simulink model "ScriptDemo"  (R2022b)
settings: configuration reference "TmVcThermal_Configuration_sub" (kept outside this file)
undefined symbols (not defined in the file): aaaa, bbbb, cTmComprCtrl_D_u8HvacFlowTable_db, cTmComprCtrl_D_u8HvacFlowTable_sw, cTmComprCtrl_n_i16ChillCmpIMax, cTmComprCtrl_n_i16ChillCmpIMin, cTmComprCtrl_n_i16ChillCmpIMin666, cTmComprCtrl_n_i16ChillCmpPMax, cTmComprCtrl_n_i16ChillCmpPMin, cTmComprCtrl_n_i16CmpChillCoolRpmKiMax, cTmComprCtrl_n_i16CmpChillCoolRpmKiMin, cTmComprCtrl_n_i16CmpChillCoolRpmKpMax, cTmComprCtrl_n_i16CmpChillCoolRpmKpMin, cTmComprCtrl_n_i16CmpCoolRpmKiMax, cTmComprCtrl_n_i16CmpCoolRpmKiMin, cTmComprCtrl_n_i16CmpCoolRpmKpMax, cTmComprCtrl_n_i16CmpCoolRpmKpMin, cTmComprCtrl_n_i16SM4CmpHeatKiMax, cTmComprCtrl_n_i16SM4CmpHeatKiMin, cTmComprCtrl_n_i16SM4CmpHeatKpMax, cTmComprCtrl_n_i16SM4CmpHeatKpMin, cTmComprCtrl_n_i16SM5CmpHeatKiMax, cTmComprCtrl_n_i16SM5CmpHeatKiMin, cTmComprCtrl_n_i16SM5CmpHeatKpMax, cTmComprCtrl_n_i16SM5CmpHeatKpMin, cTmComprCtrl_n_i16SM6CmpHeatKiMax, cTmComprCtrl_n_i16SM6CmpHeatKiMin, cTmComprCtrl_n_i16SM6CmpHeatKpMax, cTmComprCtrl_n_i16SM6CmpHeatKpMin, cTmComprCtrl_n_u16CmpMaxSpdFanFltLimt, cTmComprCtrl_n_u16CmpMaxSpdLoSidePFltLimt, cTmComprCtrl_n_u16CmpMaxSpdSensorFltLimt, cTmComprCtrl_n_u16CompMinRpm, cTmComprCtrl_n_u16CompRpmIncThres, cTmComprCtrl_t_u16BattCooltFFPeriod, cTmComprCtrl_t_u16BattCooltPIPeriod, cTmComprCtrl_t_u16CmpCoolFFPeriod, cTmComprCtrl_t_u16CmpCoolPIPeriod, cTmComprCtrl_t_u16CoolCmpChillFFPeriod, cTmComprCtrl_t_u16CoolCmpChillPIPeriod, cTmComprCtrl_t_u16SM4CmpHeatFFPeriod, cTmComprCtrl_t_u16SM4CmpHeatPIPeriod, cTmComprCtrl_t_u16SM5CmpHeatFFPeriod, cTmComprCtrl_t_u16SM5CmpHeatPIPeriod, cTmComprCtrl_t_u16SM6CmpHeatFFPeriod, cTmComprCtrl_t_u16SM6CmpHeatPIPeriod, cTmComprCtrl_Te_EvapClearInteg, cTmComprCtrl_Te_i16HpReqTempSaturoffset, cTmComprCtrl_Te_i16SatLpReplaceDiff, cTmComprCtrl_Te_i16SM3BatDiffStartEvapDecOffset, cTmComprCtrl_Te_i16SM3EvapLo, cTmComprCtrl_Te_i16SM3TBatDiffEntEvapDecOffset, cTmComprCtrl_Te_i16SM3TBatDiffEntEvapDecOffsetQuit, cTmComprCtrl_Te_s32ErrCmpChillPIContinueCoolH, cTmComprCtrl_Te_s32ErrCmpChillPIContinueCoolL, cTmComprCtrl_Te_s32ErrCmpPIContinueChillH, cTmComprCtrl_Te_s32ErrCmpPIContinueChillL, cTmComprCtrl_Te_s32ErrCmpPIContinueCoolH, cTmComprCtrl_Te_s32ErrCmpPIContinueCoolL, cTmComprCtrl_Te_s32ErrCmpPIContinueHeatH ... (+398)
libraries: simulink x782, PCMULib x640, simulink_need_slupdate x4
(part 14 of 41)

== system ScriptDemo/Create/createMerge/Before/ID29332_RpmPI ==
  note: 测试步骤：
      | 使能测试
      | 清I测试
      | 	不使能
      | 	模式切换
      | 保持I测试
      | 	上限保持
      | 	下限保持
      | 	边界限制清I保持
      | 累计限值
      | 	累计Kp, Ki 上限
      | 	累计Kp, Ki 下限
      | 正常PI测试
      | 	上升
      | 	下降
  rTmComprCtrl_Te_s32LowErrStop : Inport  OutDataTypeStr=single
  rTmComprCtrl_Te_s32TempError : Inport  Port=2  OutDataTypeStr=single
  rTmComprCtrl_Te_s32UpErrStop : Inport  Port=3  OutDataTypeStr=single
  rTmComprCtrl_n_u16ComprRpmFF : Inport  Port=4  OutDataTypeStr=uint16
  rTmComprCtrl_n_u16ComprRpmKi : Inport  Port=5  OutDataTypeStr=uint16
  rTmComprCtrl_n_u16ComprRpmKp : Inport  Port=6  OutDataTypeStr=uint16
  rTmComprCtrl_n_u16DisOverrideValue : Inport  Port=7  OutDataTypeStr=uint16
  rTmComprCtrl_n_i16KiLowLimit : Inport  Port=8  OutDataTypeStr=int16
  rTmComprCtrl_n_i16KiUpLimit : Inport  Port=9  OutDataTypeStr=int16
  rTmComprCtrl_n_i16KpLowLimit : Inport  Port=10  OutDataTypeStr=int16
  rTmComprCtrl_n_i16KpUpLimit : Inport  Port=11  OutDataTypeStr=int16
  rTmComprCtrl_t_u16PIPeriod : Inport  Port=12  OutDataTypeStr=uint16
  xTmComprCtrl_B_CompOnReqCompOn : Inport  Port=13  OutDataTypeStr=boolean
  xTmComprCtrl_B_Enable : Inport  Port=14  OutDataTypeStr=boolean
  xTmComprCtrl_B_ModeChanged : Inport  Port=15  OutDataTypeStr=boolean
  xTmComprCtrl_B_ReduceRpm : Inport  Port=16  OutDataTypeStr=boolean
  sTmRefriModeMgr_D_u8HPCurMode : Inport  Port=17  OutDataTypeStr=uint8
  sTmSigProces_Te_s32EvapFanFilter : Inport  Port=18  OutDataTypeStr=single
  yTmRefriModeMgr_B_CoolModeInCycle : Inport  Port=19  OutDataTypeStr=boolean
  yTmRefriModeMgr_B_HeatModeInCycle : Inport  Port=20  OutDataTypeStr=boolean
  ClearInteg : Subsystem  TreatAsAtomicUnit=on
  IndebugRvs : PCMULib/Interface/IndebugRvs  SWI=cTmComprCtrl_Te_s32LowErrStop_swi  DBI=cTmComprCtrl_Te_s32LowErrStop_dbi
      settings: SourceProductName=PCMULib
  IndebugRvs1 : PCMULib/Interface/IndebugRvs  SWI=cTmComprCtrl_Te_s32TempError_swi  DBI=cTmComprCtrl_Te_s32TempError_dbi
      settings: SourceProductName=PCMULib
  IndebugRvs10 : PCMULib/Interface/IndebugRvs  SWI=cTmComprCtrl_n_i16KpUpLimit_swi  DBI=cTmComprCtrl_n_i16KpUpLimit_dbi
      settings: SourceProductName=PCMULib
  IndebugRvs11 : PCMULib/Interface/IndebugRvs  SWI=cTmComprCtrl_t_u16PIPeriod_swi  DBI=cTmComprCtrl_t_u16PIPeriod_dbi
      settings: SourceProductName=PCMULib
  IndebugRvs12 : PCMULib/Interface/IndebugRvs  SWI=cTmComprCtrl_B_Enable_swi  DBI=cTmComprCtrl_B_Enable_dbi
      settings: SourceProductName=PCMULib
  IndebugRvs13 : PCMULib/Interface/IndebugRvs  SWI=cTmComprCtrl_B_ModeChanged_swi  DBI=cTmComprCtrl_B_ModeChanged_dbi
      settings: SourceProductName=PCMULib
  IndebugRvs2 : PCMULib/Interface/IndebugRvs  SWI=cTmComprCtrl_Te_s32UpErrStop_swi  DBI=cTmComprCtrl_Te_s32UpErrStop_dbi
      settings: SourceProductName=PCMULib
  IndebugRvs3 : PCMULib/Interface/IndebugRvs  SWI=cTmComprCtrl_n_u16ComprRpmFF_swi  DBI=cTmComprCtrl_n_u16ComprRpmFF_dbi
      settings: SourceProductName=PCMULib
  IndebugRvs4 : PCMULib/Interface/IndebugRvs  SWI=cTmComprCtrl_n_u16ComprRpmKi_swi  DBI=cTmComprCtrl_n_u16ComprRpmKi_dbi
      settings: SourceProductName=PCMULib
  IndebugRvs5 : PCMULib/Interface/IndebugRvs  SWI=cTmComprCtrl_n_u16ComprRpmKp_swi  DBI=cTmComprCtrl_n_u16ComprRpmKp_dbi
      settings: SourceProductName=PCMULib
  IndebugRvs6 : PCMULib/Interface/IndebugRvs  SWI=cTmComprCtrl_n_u16DisOverrideValue_swi  DBI=cTmComprCtrl_n_u16DisOverrideValue_dbi
      settings: SourceProductName=PCMULib
  IndebugRvs7 : PCMULib/Interface/IndebugRvs  SWI=cTmComprCtrl_n_i16KiLowLimit_swi  DBI=cTmComprCtrl_n_i16KiLowLimit_dbi
      settings: SourceProductName=PCMULib
  IndebugRvs8 : PCMULib/Interface/IndebugRvs  SWI=cTmComprCtrl_n_i16KiUpLimit_swi  DBI=cTmComprCtrl_n_i16KiUpLimit_dbi
      settings: SourceProductName=PCMULib
  IndebugRvs9 : PCMULib/Interface/IndebugRvs  SWI=cTmComprCtrl_n_i16KpLowLimit_swi  DBI=cTmComprCtrl_n_i16KpLowLimit_dbi
      settings: SourceProductName=PCMULib
  PIControler : Subsystem  AncestorBlock=PCMULib/Calculation/PI
  rTmComprCtrl_n_u16CompRpmReqPI : Outport  OutDataTypeStr=uint16
  wires:
  [rTmComprCtrl_t_u16PIPeriod] -> PIControler/3(rTmComprCtrl_t_u16PIPeriod)
  [rTmComprCtrl_Te_s32TempError] -> PIControler/4(rTmComprCtrl_Te_s32TempError)
  [rTmComprCtrl_n_u16ComprRpmFF] -> PIControler/5(rTmComprCtrl_n_u16ComprRpmFF)
  [rTmComprCtrl_n_u16ComprRpmKp] -> PIControler/6(rTmComprCtrl_n_u16ComprRpmKp)
  [rTmComprCtrl_n_u16ComprRpmKi] -> PIControler/7(rTmComprCtrl_n_u16ComprRpmKi)
  [rTmComprCtrl_n_i16KpLowLimit] -> PIControler/9(rTmComprCtrl_n_i16KpLowLimit)
  [rTmComprCtrl_n_i16KiUpLimit] -> PIControler/10(rTmComprCtrl_n_i16KiUpLimit)
  [rTmComprCtrl_n_i16KiLowLimit] -> PIControler/11(rTmComprCtrl_n_i16KiLowLimit)
  [rTmComprCtrl_Te_s32UpErrStop] -> PIControler/12(rTmComprCtrl_Te_s32UpErrStop)
  [rTmComprCtrl_Te_s32LowErrStop] -> PIControler/13(rTmComprCtrl_Te_s32LowErrStop)
  [rTmComprCtrl_n_u16DisOverrideValue] -> PIControler/14(rTmComprCtrl_n_u16DisOverrideValue)
  PIControler/1(rPIControler_n_u16CompRpmReq) -> [rPIControler_n_u16CompRpmReq]
  rTmComprCtrl_Te_s32LowErrStop/1 -> IndebugRvs/1
  rTmComprCtrl_Te_s32TempError/1 -> IndebugRvs1/1
  rTmComprCtrl_Te_s32UpErrStop/1 -> IndebugRvs2/1
  rTmComprCtrl_n_u16ComprRpmFF/1 -> IndebugRvs3/1
  rTmComprCtrl_n_u16ComprRpmKi/1 -> IndebugRvs4/1
  rTmComprCtrl_n_u16ComprRpmKp/1 -> IndebugRvs5/1
  rTmComprCtrl_n_u16DisOverrideValue/1 -> IndebugRvs6/1
  rTmComprCtrl_n_i16KiLowLimit/1 -> IndebugRvs7/1
  rTmComprCtrl_n_i16KiUpLimit/1 -> IndebugRvs8/1
  rTmComprCtrl_n_i16KpLowLimit/1 -> IndebugRvs9/1
  rTmComprCtrl_n_i16KpUpLimit/1 -> IndebugRvs10/1
  rTmComprCtrl_t_u16PIPeriod/1 -> IndebugRvs11/1
  xTmComprCtrl_B_CompOnReqCompOn/1 -> [xTmComprCtrl_B_CompOnReqCompOn]
  [rPIControler_n_u16CompRpmReq] -> rTmComprCtrl_n_u16CompRpmReqPI/1
  xTmComprCtrl_B_Enable/1 -> IndebugRvs12/1
  xTmComprCtrl_B_ModeChanged/1 -> IndebugRvs13/1
  IndebugRvs/1 -> [rTmComprCtrl_Te_s32LowErrStop]  "rTmComprCtrl_Te_s32LowErrStop"
  IndebugRvs1/1 -> [rTmComprCtrl_Te_s32TempError]  "rTmComprCtrl_Te_s32TempError"
  IndebugRvs2/1 -> [rTmComprCtrl_Te_s32UpErrStop]  "rTmComprCtrl_Te_s32UpErrStop"
  IndebugRvs3/1 -> [rTmComprCtrl_n_u16ComprRpmFF]  "rTmComprCtrl_n_u16ComprRpmFF"
  IndebugRvs4/1 -> [rTmComprCtrl_n_u16ComprRpmKi]  "rTmComprCtrl_n_u16ComprRpmKi"
  IndebugRvs5/1 -> [rTmComprCtrl_n_u16ComprRpmKp]  "rTmComprCtrl_n_u16ComprRpmKp"
  IndebugRvs7/1 -> [rTmComprCtrl_n_i16KiLowLimit]  "rTmComprCtrl_n_i16KiLowLimit"
  IndebugRvs6/1 -> [rTmComprCtrl_n_u16DisOverrideValue]  "rTmComprCtrl_n_u16DisOverrideValue"
  IndebugRvs8/1 -> [rTmComprCtrl_n_i16KiUpLimit]  "rTmComprCtrl_n_i16KiUpLimit"
  IndebugRvs9/1 -> [rTmComprCtrl_n_i16KpLowLimit]  "rTmComprCtrl_n_i16KpLowLimit"
  IndebugRvs11/1 -> [rTmComprCtrl_t_u16PIPeriod]  "rTmComprCtrl_t_u16PIPeriod"
  IndebugRvs10/1 -> [rTmComprCtrl_n_i16KpUpLimit]  "rTmComprCtrl_n_i16KpUpLimit"
  IndebugRvs12/1 -> [xTmComprCtrl_B_Enable]  "xTmComprCtrl_B_Enable"
  IndebugRvs13/1 -> [xTmComprCtrl_B_ModeChanged]  "xTmComprCtrl_B_ModeChanged"
  xTmComprCtrl_B_ReduceRpm/1 -> [xTmComprCtrl_B_ReduceRpm]
  [xTmComprCtrl_B_ReduceRpm] -> PIControler/15(xTmComprCtrl_B_ReduceRpm)
  [rTmComprCtrl_n_i16KpUpLimit] -> PIControler/8(rTmComprCtrl_n_i16KpUpLimit)
  [xTmComprCtrl_B_Enable] -> PIControler/1(xTmComprCtrl_B_Enable)
  PIControler/2(rPIControler_n_s32SAccmKi) -> [rPIControler_n_s32SAccmKi]
  [rPIControler_n_s32SAccmKi] -> ClearInteg/1(rPIControler_n_s32SAccmKi)
  [sTmRefriModeMgr_D_u8HPCurMode] -> ClearInteg/2(sTmRefriModeMgr_D_u8HPCurMode)
  [sTmSigProces_Te_s32EvapFanFilter] -> ClearInteg/3(sTmSigProces_Te_s32EvapFanFilter)
  [xTmComprCtrl_B_CompOnReqCompOn] -> ClearInteg/4(xTmComprCtrl_B_CompOnReqCompOn)
  [xTmComprCtrl_B_ModeChanged] -> ClearInteg/5(xTmComprCtrl_B_ModeChanged)
  ClearInteg/1(xClearInteg_B_ClearInteg) -> [xClearInteg_B_ClearInteg]
  [xClearInteg_B_ClearInteg] -> PIControler/2(xTmComprCtrl_B_ClearInteg)
  sTmRefriModeMgr_D_u8HPCurMode/1 -> [sTmRefriModeMgr_D_u8HPCurMode]
  sTmSigProces_Te_s32EvapFanFilter/1 -> [sTmSigProces_Te_s32EvapFanFilter]
  [yTmRefriModeMgr_B_CoolModeInCycle] -> ClearInteg/6(yTmRefriModeMgr_B_CoolModeInCycle)
  [yTmRefriModeMgr_B_HeatModeInCycle] -> ClearInteg/7(yTmRefriModeMgr_B_HeatModeInCycle)
  yTmRefriModeMgr_B_CoolModeInCycle/1 -> [yTmRefriModeMgr_B_CoolModeInCycle]
  yTmRefriModeMgr_B_HeatModeInCycle/1 -> [yTmRefriModeMgr_B_HeatModeInCycle]

== system ScriptDemo/Create/createMerge/Before/SM0 ==
  Action Port : ActionPort
  Constant{,1..2,10} (4 alike) : Constant  Value=0  OutDataTypeStr=uint16
  Constant11 : Constant  Value=5  OutDataTypeStr=uint16
  Constant12 : Constant  Value=0  OutDataTypeStr=boolean
  Constant3 : Constant  Value=0  OutDataTypeStr=single
  Constant4 : Constant  Value=0  OutDataTypeStr=single
  Constant5 : Constant  Value=0  OutDataTypeStr=single
  Constant{6..9} (4 alike) : Constant  Value=0  OutDataTypeStr=int16
  rSM0_Te_s32TempError : Outport  OutDataTypeStr=single
  rSM0_n_u16ComprRpmFF : Outport  Port=2  OutDataTypeStr=uint16
  rSM0_n_u16DisOverrideValue : Outport  Port=3  OutDataTypeStr=uint16
  rSM0_t_u16PIPeriod : Outport  Port=4  OutDataTypeStr=uint16
  xSM0_B_Enable : Outport  Port=5  OutDataTypeStr=boolean
  rSM0_n_u16ComprRpmKp : Outport  Port=6  OutDataTypeStr=uint16
  rSM0_n_u16ComprRpmKi : Outport  Port=7  OutDataTypeStr=uint16
  rSM0_Te_s32UpErrStop : Outport  Port=8  OutDataTypeStr=single
  rSM0_Te_s32LowErrStop : Outport  Port=9  OutDataTypeStr=single
  rSM0_n_i16KpUpLimit : Outport  Port=10  OutDataTypeStr=int16
  rSM0_n_i16KpLowLimit : Outport  Port=11  OutDataTypeStr=int16
  rSM0_n_i16KiUpLimit : Outport  Port=12  OutDataTypeStr=int16
  rSM0_n_i16KiLowLimit : Outport  Port=13  OutDataTypeStr=int16
  wires:
  Constant/1 -> [rTmComprCtrl_n_u16ComprRpmFF]
  Constant1/1 -> [rTmComprCtrl_n_u16ComprRpmKp]
  Constant2/1 -> [rTmComprCtrl_n_u16ComprRpmKi]
  Constant4/1 -> [rTmComprCtrl_Te_s32TempError]
  Constant3/1 -> [rTmComprCtrl_Te_s32UpErrStop]
  Constant5/1 -> [rTmComprCtrl_Te_s32LowErrStop]
  Constant6/1 -> [rTmComprCtrl_n_i16KpUpLimit]
  Constant7/1 -> [rTmComprCtrl_n_i16KpLowLimit]
  Constant8/1 -> [rTmComprCtrl_n_i16KiUpLimit]
  Constant9/1 -> [rTmComprCtrl_n_i16KiLowLimit]
  Constant10/1 -> [rTmComprCtrl_n_u16DisOverrideValue]
  Constant11/1 -> [rTmComprCtrl_t_u16PIPeriod]
  Constant12/1 -> [xTmComprCtrl_B_Enable]
  [rTmComprCtrl_Te_s32TempError] -> rSM0_Te_s32TempError/1
  [rTmComprCtrl_n_u16ComprRpmFF] -> rSM0_n_u16ComprRpmFF/1
  [rTmComprCtrl_n_u16DisOverrideValue] -> rSM0_n_u16DisOverrideValue/1
  [rTmComprCtrl_t_u16PIPeriod] -> rSM0_t_u16PIPeriod/1
  [xTmComprCtrl_B_Enable] -> xSM0_B_Enable/1
  [rTmComprCtrl_n_u16ComprRpmKp] -> rSM0_n_u16ComprRpmKp/1
  [rTmComprCtrl_n_u16ComprRpmKi] -> rSM0_n_u16ComprRpmKi/1
  [rTmComprCtrl_Te_s32UpErrStop] -> rSM0_Te_s32UpErrStop/1
  [rTmComprCtrl_Te_s32LowErrStop] -> rSM0_Te_s32LowErrStop/1
  [rTmComprCtrl_n_i16KpUpLimit] -> rSM0_n_i16KpUpLimit/1
  [rTmComprCtrl_n_i16KpLowLimit] -> rSM0_n_i16KpLowLimit/1
  [rTmComprCtrl_n_i16KiUpLimit] -> rSM0_n_i16KiUpLimit/1
  [rTmComprCtrl_n_i16KiLowLimit] -> rSM0_n_i16KiLowLimit/1

== system ScriptDemo/Create/createMerge/Before/SM1SM21 ==
  sTmIn_D_u8DCChrgSt : Inport  OutDataTypeStr=uint8
  sTmIn_Te_s32HvBattCooltTReq : Inport  Port=2  OutDataTypeStr=single
  sTmSigProces_D_u8BattThermReq : Inport  Port=3  OutDataTypeStr=uint8
  sTmSigProces_D_u8HvBattCoolgReq : Inport  Port=4  OutDataTypeStr=uint8
  sTmSigProces_Te_s32HvBattCooltTFilter : Inport  Port=5  OutDataTypeStr=single
  xTmComprCtrl_B_CompOnReqCompOn : Inport  Port=6  OutDataTypeStr=boolean
  sTmSigProces_Te_s32TAmb : Inport  Port=7  OutDataTypeStr=single
  sTmIn_D_u8HeatPump : Inport  Port=8  OutDataTypeStr=uint8
  Action Port : ActionPort
  Constant : Constant  Value=cTmComprCtrl_n_i16ChillCmpPMax  OutDataTypeStr=int16
  Constant1 : Constant  Value=cTmComprCtrl_t_u16BattCooltPIPeriod  OutDataTypeStr=uint16
  Constant10 : Constant  Value=0  OutDataTypeStr=uint16
  Constant12 : Constant  OutDataTypeStr=boolean
  Constant2 : Constant  Value=cTmComprCtrl_n_i16ChillCmpPMin  OutDataTypeStr=int16
  Constant3 : Constant  Value=cTmComprCtrl_Te_s32ErrCmpPIContinueChillH  OutDataTypeStr=single
  Constant4 : Constant  Value=cTmComprCtrl_n_i16ChillCmpIMax  OutDataTypeStr=int16
  Constant5 : Constant  Value=cTmComprCtrl_Te_s32ErrCmpPIContinueChillL  OutDataTypeStr=single
  Constant6 : Constant  Value=cTmComprCtrl_n_i16ChillCmpIMin  OutDataTypeStr=int16
  ID26245_SM1FF : Subsystem
  ID26247_SM1Error : Subsystem
  SM1FFEnable : Subsystem
  SM1_Ki : Subsystem
  SM1_Kp : Subsystem
  rSM1SM21_n_u16DisOverrideValue : Outport  OutDataTypeStr=uint16
  rSM1SM21_t_u16PIPeriod : Outport  Port=2  OutDataTypeStr=uint16
  rSM1SM21_Te_s32UpErrStop : Outport  Port=3  OutDataTypeStr=single
  rSM1SM21_Te_s32LowErrStop : Outport  Port=4  OutDataTypeStr=single
  rSM1SM21_n_i16KpUpLimit : Outport  Port=5  OutDataTypeStr=int16
  rSM1SM21_n_u16ComprRpmFF : Outport  Port=6  OutDataTypeStr=uint16
  rSM1SM21_n_u16ComprRpmKp : Outport  Port=7  OutDataTypeStr=uint16
  rSM1SM21_n_u16ComprRpmKi : Outport  Port=8  OutDataTypeStr=uint16
  rSM1SM21_n_i16KpLowLimit : Outport  Port=9  OutDataTypeStr=int16
  rSM1SM21_n_i16KiUpLimit : Outport  Port=10  OutDataTypeStr=int16
  rSM1SM21_n_i16KiLowLimit : Outport  Port=11  OutDataTypeStr=int16
  xSM1SM21_B_Enable : Outport  Port=12  OutDataTypeStr=boolean
  rSM1SM21_Te_s32TempError : Outport  Port=13  OutDataTypeStr=single
  wires:
  ID26247_SM1Error/1(rTmComprCtrl_Te_s32TempError) -> [rTmComprCtrl_Te_s32TempError]
  [sTmIn_Te_s32HvBattCooltTReq] -> ID26247_SM1Error/1(sTmIn_Te_s32HvBattCooltTReq)
  [sTmSigProces_Te_s32HvBattCooltTFilter] -> ID26247_SM1Error/2(sTmSigProces_Te_s32HvBattCooltTFilter)
  [sTmSigProces_D_u8BattThermReq] -> SM1_Kp/1(sTmSigProces_D_u8BattThermReq)
  [sTmIn_D_u8DCChrgSt] -> SM1_Kp/2(sTmIn_D_u8DCChrgSt)
  [sTmSigProces_D_u8HvBattCoolgReq] -> SM1_Kp/3(sTmSigProces_D_u8HvBattCoolgReq)
  [rTmComprCtrl_Te_s32TempError] -> SM1_Kp/4(rTmComprCtrl_Te_s32TempError)
  [sTmSigProces_D_u8BattThermReq] -> SM1_Ki/1(sTmSigProces_D_u8BattThermReq)
  [sTmIn_D_u8DCChrgSt] -> SM1_Ki/2(sTmIn_D_u8DCChrgSt)
  [sTmSigProces_D_u8HvBattCoolgReq] -> SM1_Ki/3(sTmSigProces_D_u8HvBattCoolgReq)
  [rTmComprCtrl_Te_s32TempError] -> SM1_Ki/4(rTmComprCtrl_Te_s32TempError)
  [sTmIn_Te_s32HvBattCooltTReq] -> ID26245_SM1FF/1(sTmIn_Te_s32HvBattCooltTReq)
  [sTmIn_D_u8DCChrgSt] -> ID26245_SM1FF/2(sTmIn_D_u8DCChrgSt)
  [sTmSigProces_D_u8HvBattCoolgReq] -> ID26245_SM1FF/3(sTmSigProces_D_u8HvBattCoolgReq)
  [xTmComprCtrl_B_CompOnReqCompOn] -> SM1FFEnable/1(xTmComprCtrl_B_CompOnReqCompOn)
  SM1FFEnable/1(SM1FFEnable_B_SM1FFEnable) -> [SM1FFEnable_B_SM1FFEnable]
  [SM1FFEnable_B_SM1FFEnable] -> ID26245_SM1FF/Enable
  SM1_Ki/1(SM1Ki) -> [rTmComprCtrl_n_u16ComprRpmKi]
  SM1_Kp/1(SM1Kp) -> [rTmComprCtrl_n_u16ComprRpmKp]
  ID26245_SM1FF/1(SM1FF) -> [rTmComprCtrl_n_u16ComprRpmFF]
  sTmIn_D_u8DCChrgSt/1 -> [sTmIn_D_u8DCChrgSt]
  sTmIn_Te_s32HvBattCooltTReq/1 -> [sTmIn_Te_s32HvBattCooltTReq]
  sTmSigProces_D_u8BattThermReq/1 -> [sTmSigProces_D_u8BattThermReq]
  sTmSigProces_D_u8HvBattCoolgReq/1 -> [sTmSigProces_D_u8HvBattCoolgReq]
  sTmSigProces_Te_s32HvBattCooltTFilter/1 -> [sTmSigProces_Te_s32HvBattCooltTFilter]
  xTmComprCtrl_B_CompOnReqCompOn/1 -> [xTmComprCtrl_B_CompOnReqCompOn]
  Constant10/1 -> [rTmComprCtrl_n_u16DisOverrideValue]
  Constant4/1 -> [rTmComprCtrl_n_i16KiUpLimit]
  Constant6/1 -> [rTmComprCtrl_n_i16KiLowLimit]
  Constant1/1 -> [rTmComprCtrl_t_u16PIPeriod]
  Constant5/1 -> [rTmComprCtrl_Te_s32LowErrStop]
  Constant2/1 -> [rTmComprCtrl_n_i16KpLowLimit]
  Constant/1 -> [rTmComprCtrl_n_i16KpUpLimit]
  Constant3/1 -> [rTmComprCtrl_Te_s32UpErrStop]
  Constant12/1 -> [xTmComprCtrl_B_Enable]
  [sTmSigProces_Te_s32TAmb] -> ID26245_SM1FF/4(sTmSigProces_Te_s32TAmb)
  sTmSigProces_Te_s32TAmb/1 -> [sTmSigProces_Te_s32TAmb]
  [sTmIn_D_u8HeatPump] -> ID26245_SM1FF/5(sTmIn_D_u8HeatPump)
  sTmIn_D_u8HeatPump/1 -> [sTmIn_D_u8HeatPump]
  [rTmComprCtrl_n_u16DisOverrideValue] -> rSM1SM21_n_u16DisOverrideValue/1
  [rTmComprCtrl_t_u16PIPeriod] -> rSM1SM21_t_u16PIPeriod/1
  [rTmComprCtrl_Te_s32UpErrStop] -> rSM1SM21_Te_s32UpErrStop/1
  [rTmComprCtrl_Te_s32LowErrStop] -> rSM1SM21_Te_s32LowErrStop/1
  [rTmComprCtrl_n_i16KpUpLimit] -> rSM1SM21_n_i16KpUpLimit/1
  [rTmComprCtrl_n_u16ComprRpmFF] -> rSM1SM21_n_u16ComprRpmFF/1
  [rTmComprCtrl_n_u16ComprRpmKp] -> rSM1SM21_n_u16ComprRpmKp/1
  [rTmComprCtrl_n_u16ComprRpmKi] -> rSM1SM21_n_u16ComprRpmKi/1
  [rTmComprCtrl_n_i16KpLowLimit] -> rSM1SM21_n_i16KpLowLimit/1
  [rTmComprCtrl_n_i16KiUpLimit] -> rSM1SM21_n_i16KiUpLimit/1
  [rTmComprCtrl_n_i16KiLowLimit] -> rSM1SM21_n_i16KiLowLimit/1
  [xTmComprCtrl_B_Enable] -> xSM1SM21_B_Enable/1
  [rTmComprCtrl_Te_s32TempError] -> rSM1SM21_Te_s32TempError/1

== system ScriptDemo/Create/createMerge/Before/SM2SM22 ==
  note: 1: 非热泵
      | 2：热泵
  sTmSigProces_Te_s32EvapFanReqRamp : Inport  OutDataTypeStr=single
  sTmDiag_D_u8TeEvapFltSt : Inport  Port=2  OutDataTypeStr=uint8
  sTmIn_D_u8HeatPump : Inport  Port=3  OutDataTypeStr=uint8
  sTmSigProces_Te_s32TAmb : Inport  Port=4  OutDataTypeStr=single
  sTmIn_X_s32ClimtRcirc : Inport  Port=5  OutDataTypeStr=single
  sTmComprCtrl_D_u8HvacFlowLevel : Inport  Port=6  OutDataTypeStr=uint8
  sTmSigProces_Te_s32EvapFanFilter : Inport  Port=7  OutDataTypeStr=single
  sTmSigProces_Te_s32SatLp : Inport  Port=8  OutDataTypeStr=single
  xTmComprCtrl_B_CompOnReqCompOn : Inport  Port=9  OutDataTypeStr=boolean
  yTmRefriModeMgr_B_CoolModeInCycle : Inport  Port=10  OutDataTypeStr=boolean
  yTmRefriModeMgr_B_CoolOCRMode : Inport  Port=11  OutDataTypeStr=boolean
  sTmSigProces_Pw_i16ReqPwrForCool : Inport  Port=12  OutDataTypeStr=int16
  Action Port : ActionPort
  1-D Lookup Table : Lookup_n-D  NumberOfTableDimensions=1  BreakpointsForDimension1=tTmComprCtrl_n_i16CmpCoolRpmKiMin_X  BreakpointsForDimension1DataTypeStr=Inherit: Inherit from 'Breakpoint data'  Table=tTmComprCtrl_n_i16CmpCoolRpmKiMin  TableDataTypeStr=Inherit: Inherit from 'Table data'  ExtrapMethod=Clip  InternalRulePriority=Speed  OutDataTypeStr=Inherit: Inherit via back propagation  RndMeth=Simplest  InputSameDT=off
  1-D Lookup Table1 : Lookup_n-D  NumberOfTableDimensions=1  BreakpointsForDimension1=tTmComprCtrl_n_i16CmpCoolRpmKiMax_X  BreakpointsForDimension1DataTypeStr=Inherit: Inherit from 'Breakpoint data'  Table=tTmComprCtrl_n_i16CmpCoolRpmKiMax  TableDataTypeStr=Inherit: Inherit from 'Table data'  ExtrapMethod=Clip  InternalRulePriority=Speed  OutDataTypeStr=Inherit: Inherit via back propagation  RndMeth=Simplest  InputSameDT=off
  Compare To Constant1 : simulink/Logic and Bit Operations/Compare To Constant  relop===  const=2  OutDataTypeStr=boolean
  Constant : Constant  Value=cTmComprCtrl_n_i16CmpCoolRpmKpMax  OutDataTypeStr=int16
  Constant3 : Constant  Value=cTmComprCtrl_t_u16CmpCoolPIPeriod  OutDataTypeStr=uint16
  Constant4 : Constant  Value=cTmComprCtrl_n_i16CmpCoolRpmKpMin  OutDataTypeStr=int16
  Constant5 : Constant  Value=cTmComprCtrl_Te_s32ErrCmpPIContinueCoolH  OutDataTypeStr=single
  Constant6 : Constant  Commented=on  Value=cTmComprCtrl_n_i16CmpCoolRpmKiMax  OutDataTypeStr=int16
  Constant7 : Constant  Value=cTmComprCtrl_Te_s32ErrCmpPIContinueCoolL  OutDataTypeStr=single
  Constant8 : Constant  Commented=on  Value=cTmComprCtrl_n_i16CmpCoolRpmKiMin  OutDataTypeStr=int16
  Constant9 : Constant  Value=cTmComprCtrl_n_u16CompMinRpm
  ID26239_SM2Error : Subsystem
  ID26267_SM2FF : Subsystem
  Logical Operator : Logic  AllPortsSameDT=off  OutDataTypeStr=boolean
  Logical Operator2 : Logic  Operator=NOT  AllPortsSameDT=off  OutDataTypeStr=boolean
  SM2FFEnable : Subsystem
  SM2_Ki : Subsystem
  SM2_Kp : Subsystem
  rSM2SM22_n_u16DisOverrideValue : Outport  OutDataTypeStr=uint16
  rSM2SM22_t_u16PIPeriod : Outport  Port=2  OutDataTypeStr=uint16
  rSM2SM22_Te_s32UpErrStop : Outport  Port=3  OutDataTypeStr=single
  rSM2SM22_n_u16ComprRpmFF : Outport  Port=4  OutDataTypeStr=uint16
  rSM2SM22_n_u16ComprRpmKp : Outport  Port=5  OutDataTypeStr=uint16
  rSM2SM22_n_u16ComprRpmKi : Outport  Port=6  OutDataTypeStr=uint16
  rSM2SM22_Te_s32LowErrStop : Outport  Port=7  OutDataTypeStr=single
  rSM2SM22_n_i16KpUpLimit : Outport  Port=8  OutDataTypeStr=int16
  rSM2SM22_n_i16KpLowLimit : Outport  Port=9  OutDataTypeStr=int16
  rSM2SM22_n_i16KiUpLimit : Outport  Port=10  OutDataTypeStr=int16
  rSM2SM22_n_i16KiLowLimit : Outport  Port=11  OutDataTypeStr=int16
  xSM2SM22_B_Enable : Outport  Port=12  OutDataTypeStr=boolean
  rSM2SM22_Te_s32TempError : Outport  Port=13  OutDataTypeStr=single
  wires:
  sTmSigProces_Te_s32EvapFanReqRamp/1 -> [sTmSigProces_Te_s32EvapFanReqRamp]
  sTmDiag_D_u8TeEvapFltSt/1 -> [sTmDiag_D_u8TeEvapFltSt]
  sTmIn_D_u8HeatPump/1 -> [sTmIn_D_u8HeatPump]
  sTmSigProces_Te_s32TAmb/1 -> [sTmSigProces_Te_s32TAmb]
  sTmIn_X_s32ClimtRcirc/1 -> [sTmIn_X_s32ClimtRcirc]
  sTmComprCtrl_D_u8HvacFlowLevel/1 -> [sTmComprCtrl_D_u8HvacFlowLevel]
  sTmSigProces_Te_s32EvapFanFilter/1 -> [sTmSigProces_Te_s32EvapFanFilter]
  sTmSigProces_Te_s32SatLp/1 -> [sTmSigProces_Te_s32SatLp]
  xTmComprCtrl_B_CompOnReqCompOn/1 -> [xTmComprCtrl_B_CompOnReqCompOn]
  yTmRefriModeMgr_B_CoolModeInCycle/1 -> [yTmRefriModeMgr_B_CoolModeInCycle]
  [sTmSigProces_Te_s32EvapFanReqRamp] -> ID26267_SM2FF/1(sTmSigProces_Te_s32EvapFanReqRamp)
  [sTmSigProces_Te_s32TAmb] -> ID26267_SM2FF/2(sTmSigProces_Te_s32TAmb)
  [sTmIn_X_s32ClimtRcirc] -> ID26267_SM2FF/3(sTmIn_X_s32ClimtRcirc)
  [sTmComprCtrl_D_u8HvacFlowLevel] -> ID26267_SM2FF/4(sTmComprCtrl_D_u8HvacFlowLevel)
  [rTmComprCtrl_Te_s32TempError] -> SM2_Ki/1(rTmComprCtrl_Te_s32TempError)
  [sTmSigProces_Te_s32TAmb] -> SM2_Ki/2(sTmSigProces_Te_s32TAmb)
  [sTmIn_X_s32ClimtRcirc] -> SM2_Ki/3(sTmIn_X_s32ClimtRcirc)
  [sTmComprCtrl_D_u8HvacFlowLevel] -> SM2_Ki/4(sTmComprCtrl_D_u8HvacFlowLevel)
  [rTmComprCtrl_Te_s32TempError] -> SM2_Kp/1(rTmComprCtrl_Te_s32TempError)
  [sTmSigProces_Te_s32TAmb] -> SM2_Kp/2(sTmSigProces_Te_s32TAmb)
  [sTmIn_X_s32ClimtRcirc] -> SM2_Kp/3(sTmIn_X_s32ClimtRcirc)
  [sTmComprCtrl_D_u8HvacFlowLevel] -> SM2_Kp/4(sTmComprCtrl_D_u8HvacFlowLevel)
  [sTmSigProces_Te_s32EvapFanReqRamp] -> ID26239_SM2Error/1(sTmSigProces_Te_s32EvapFanReqRamp)
  [sTmDiag_D_u8TeEvapFltSt] -> ID26239_SM2Error/2(sTmDiag_D_u8TeEvapFltSt)
  [sTmSigProces_Te_s32EvapFanFilter] -> ID26239_SM2Error/3(sTmSigProces_Te_s32EvapFanFilter)
  [sTmSigProces_Te_s32SatLp] -> ID26239_SM2Error/4(sTmSigProces_Te_s32SatLp)
  SM2FFEnable/1(SM2FFEnable_B_SM2FFEnable) -> [SM2FFEnable_B_SM2FFEnable]
  [xTmComprCtrl_B_CompOnReqCompOn] -> SM2FFEnable/1(xTmComprCtrl_B_CompOnReqCompOn)
  [SM2FFEnable_B_SM2FFEnable] -> ID26267_SM2FF/Enable
  ID26239_SM2Error/1(rTmComprCtrl_Te_s32TempError) -> [rTmComprCtrl_Te_s32TempError]
  ID26267_SM2FF/1(SM2FF) -> [rTmComprCtrl_n_u16ComprRpmFF]
  SM2_Kp/1(SM2Kp) -> [rTmComprCtrl_n_u16ComprRpmKp]
  SM2_Ki/1(SM2Ki) -> [rTmComprCtrl_n_u16ComprRpmKi]
  Constant9/1 -> [rTmComprCtrl_n_u16DisOverrideValue]
  Constant5/1 -> [rTmComprCtrl_Te_s32UpErrStop]
  Constant7/1 -> [rTmComprCtrl_Te_s32LowErrStop]
  Constant3/1 -> [rTmComprCtrl_t_u16PIPeriod]
  Constant/1 -> [rTmComprCtrl_n_i16KpUpLimit]
  Logical Operator/1 -> Logical Operator2/1
  [sTmIn_D_u8HeatPump] -> Compare To Constant1/1
  Compare To Constant1/1 -> Logical Operator/1
  [yTmRefriModeMgr_B_CoolModeInCycle] -> Logical Operator/2
  Logical Operator2/1 -> [xTmComprCtrl_B_Enable]
  [yTmRefriModeMgr_B_CoolOCRMode] -> ID26239_SM2Error/5(yTmRefriModeMgr_B_CoolOCRMode)
  yTmRefriModeMgr_B_CoolOCRMode/1 -> [yTmRefriModeMgr_B_CoolOCRMode]
  [sTmIn_D_u8HeatPump] -> ID26267_SM2FF/5(sTmIn_D_u8HeatPump)
  [sTmSigProces_Pw_i16ReqPwrForCool] -> 1-D Lookup Table/1, 1-D Lookup Table1/1
  Constant4/1 -> [rTmComprCtrl_n_i16KpLowLimit]
  1-D Lookup Table1/1 -> [rTmComprCtrl_n_i16KiUpLimit]
  1-D Lookup Table/1 -> [rTmComprCtrl_n_i16KiLowLimit]
  sTmSigProces_Pw_i16ReqPwrForCool/1 -> [sTmSigProces_Pw_i16ReqPwrForCool]
  [rTmComprCtrl_n_u16DisOverrideValue] -> rSM2SM22_n_u16DisOverrideValue/1
  [rTmComprCtrl_t_u16PIPeriod] -> rSM2SM22_t_u16PIPeriod/1
  [rTmComprCtrl_Te_s32UpErrStop] -> rSM2SM22_Te_s32UpErrStop/1
  [rTmComprCtrl_n_u16ComprRpmFF] -> rSM2SM22_n_u16ComprRpmFF/1
  [rTmComprCtrl_n_u16ComprRpmKp] -> rSM2SM22_n_u16ComprRpmKp/1
  [rTmComprCtrl_n_u16ComprRpmKi] -> rSM2SM22_n_u16ComprRpmKi/1
  [rTmComprCtrl_Te_s32LowErrStop] -> rSM2SM22_Te_s32LowErrStop/1
  [rTmComprCtrl_n_i16KpUpLimit] -> rSM2SM22_n_i16KpUpLimit/1
  [rTmComprCtrl_n_i16KpLowLimit] -> rSM2SM22_n_i16KpLowLimit/1
  [rTmComprCtrl_n_i16KiUpLimit] -> rSM2SM22_n_i16KiUpLimit/1
  [rTmComprCtrl_n_i16KiLowLimit] -> rSM2SM22_n_i16KiLowLimit/1
  [xTmComprCtrl_B_Enable] -> xSM2SM22_B_Enable/1
  [rTmComprCtrl_Te_s32TempError] -> rSM2SM22_Te_s32TempError/1

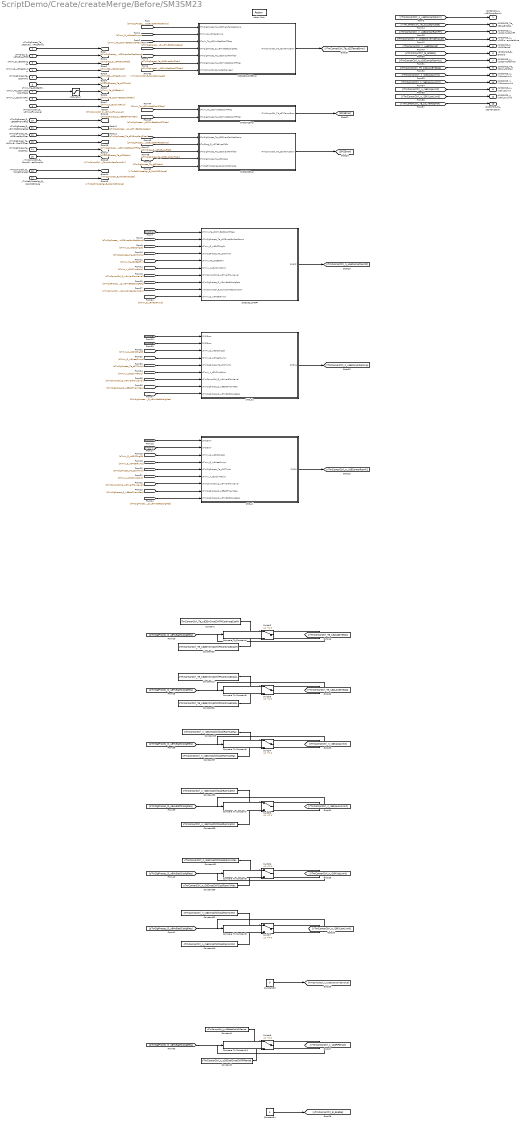
== system ScriptDemo/Create/createMerge/Before/SM3SM23 ==
  sTmSigProces_Te_s32EvapFanReqRamp : Inport  OutDataTypeStr=single
  sTmDiag_D_u8TeEvapFltSt : Inport  Port=2  OutDataTypeStr=uint8
  sTmIn_D_u8DCChrgSt : Inport  Port=3  OutDataTypeStr=uint8
  sTmIn_D_u8HeatPump : Inport  Port=4  OutDataTypeStr=uint8
  sTmSigProces_Te_s32TAmb : Inport  Port=5  OutDataTypeStr=single
  sTmIn_Te_s32BattHv : Inport  Port=6  OutDataTypeStr=single
  sTmIn_Te_s32HvBattCooltTReq : Inport  Port=7  OutDataTypeStr=single
  sTmIn_X_s32ClimtRcirc : Inport  Port=8  OutDataTypeStr=single
  sTmComprCtrl_D_u8HvacFlowLevel : Inport  Port=9  OutDataTypeStr=uint8
  sTmSigProces_D_u8BattThermReq : Inport  Port=10  OutDataTypeStr=uint8
  sTmSigProces_D_u8HvBattCoolgReq : Inport  Port=11  OutDataTypeStr=uint8
  sTmSigProces_Te_s32EvapFanFilter : Inport  Port=12  OutDataTypeStr=single
  sTmSigProces_Te_s32HvBattCooltTFilter : Inport  Port=13  OutDataTypeStr=single
  sTmSigProces_Te_s32SatLp : Inport  Port=14  OutDataTypeStr=single
  xTmComprCtrl_B_CompOnReqCompOn : Inport  Port=15  OutDataTypeStr=boolean
  xTmComprCtrl_B_ModeChanged : Inport  Port=16  OutDataTypeStr=boolean
  yTmRefriModeMgr_B_CoolOCRMode : Inport  Port=17  OutDataTypeStr=boolean
  Action Port : ActionPort
  Compare To Constant{4..9,11} (7 alike) : simulink/Logic and Bit Operations/Compare To Constant  relop===  const=3  OutDataTypeStr=boolean
  Constant : Constant  Value=cTmComprCtrl_Te_s32ErrCmpChillPIContinueCoolH  OutDataTypeStr=single
  Constant1 : Constant  Value=cTmComprCtrl_t_u16BattCooltPIPeriod  OutDataTypeStr=uint16
  Constant13 : Constant  Value=cTmComprCtrl_Te_s32ErrCmpChillPIContinueCoolL  OutDataTypeStr=single
  Constant2 : Constant  Value=cTmComprCtrl_t_u16CoolCmpChillPIPeriod  OutDataTypeStr=uint16
  Constant29 : Constant  Value=cTmComprCtrl_n_i16CmpChillCoolRpmKpMax
  Constant30 : Constant  Value=cTmComprCtrl_n_i16CmpChillCoolRpmKpMin
  Constant31 : Constant  Value=cTmComprCtrl_n_i16CmpChillCoolRpmKiMax
  Constant32 : Constant  Value=cTmComprCtrl_n_i16CmpChillCoolRpmKiMin
  Constant33 : Constant  Value=0  OutDataTypeStr=uint16
  Constant34 : Constant  OutDataTypeStr=boolean
  Constant35 : Constant  Value=cTmComprCtrl_Te_s32ErrCmpChillPIContinueCoolH  OutDataTypeStr=single
  Constant36 : Constant  Value=cTmComprCtrl_Te_s32ErrCmpChillPIContinueCoolL  OutDataTypeStr=single
  Constant37 : Constant  Value=cTmComprCtrl_n_i16CmpChillCoolRpmKpMax
  Constant38 : Constant  Value=cTmComprCtrl_n_i16CmpChillCoolRpmKpMin
  Constant39 : Constant  Value=cTmComprCtrl_n_i16CmpChillCoolRpmKiMax
  Constant40 : Constant  Value=cTmComprCtrl_n_i16CmpChillCoolRpmKiMin
  ID26262_SM3FF : Subsystem
  ID26263_SM3Error : Subsystem
  SM3SM1Error : Subsystem
  SM3SM2Error : Subsystem
  SM3_Ki : Subsystem
  SM3_Kp : Subsystem
  Saturation : Saturate  UpperLimit=40  LowerLimit=12
  Switch{2..7,9} (7 alike) : Switch  Criteria=u2 ~= 0  SaturateOnIntegerOverflow=off  InputSameDT=off
  rSM3SM23_n_u16ComprRpmKi : Outport  OutDataTypeStr=uint16
  rSM3SM23_Te_s32UpErrStop : Outport  Port=2  OutDataTypeStr=single
  rSM3SM23_n_u16ComprRpmFF : Outport  Port=3  OutDataTypeStr=uint16
  rSM3SM23_n_u16DisOverrideValue : Outport  Port=4  OutDataTypeStr=uint16
  rSM3SM23_t_u16PIPeriod : Outport  Port=5  OutDataTypeStr=uint16
  xSM3SM23_B_Enable : Outport  Port=6  OutDataTypeStr=boolean
  rSM3SM23_n_u16ComprRpmKp : Outport  Port=7  OutDataTypeStr=uint16
  rSM3SM23_Te_s32LowErrStop : Outport  Port=8  OutDataTypeStr=single
  rSM3SM23_n_i16KpUpLimit : Outport  Port=9  OutDataTypeStr=int16
  rSM3SM23_n_i16KpLowLimit : Outport  Port=10  OutDataTypeStr=int16
  rSM3SM23_n_i16KiUpLimit : Outport  Port=11  OutDataTypeStr=int16
  rSM3SM23_n_i16KiLowLimit : Outport  Port=12  OutDataTypeStr=int16
  rSM3SM23_Te_s32TempError : Outport  Port=13  OutDataTypeStr=single
  wires:
  ID26263_SM3Error/1(rTmComprCtrl_Te_s32TempError) -> [rTmComprCtrl_Te_s32TempError]
  [sTmIn_Te_s32HvBattCooltTReq] -> SM3SM1Error/1(sTmIn_Te_s32HvBattCooltTReq)
  [sTmSigProces_Te_s32HvBattCooltTFilter] -> SM3SM1Error/2(sTmSigProces_Te_s32HvBattCooltTFilter)
  [sTmDiag_D_u8TeEvapFltSt] -> SM3SM2Error/2(sTmDiag_D_u8TeEvapFltSt)
  [sTmSigProces_Te_s32EvapFanFilter] -> SM3SM2Error/3(sTmSigProces_Te_s32EvapFanFilter)
  [sTmSigProces_Te_s32SatLp] -> SM3SM2Error/4(sTmSigProces_Te_s32SatLp)
  SM3SM2Error/1(rTmComprCtrl_Te_s32TempError) -> [SM2Error]
  [sTmSigProces_Te_s32EvapFanReqRamp] -> SM3SM2Error/1(sTmSigProces_Te_s32EvapFanReqRamp)
  [SM1Error] -> SM3_Ki/1(SM1Error)
  [SM2Error] -> SM3_Ki/2(SM2Error)
  [sTmIn_D_u8DCChrgSt] -> SM3_Ki/3(sTmIn_D_u8DCChrgSt)
  [sTmIn_D_u8HeatPump] -> SM3_Ki/4(sTmIn_D_u8HeatPump)
  [sTmSigProces_Te_s32TAmb] -> SM3_Ki/5(sTmSigProces_Te_s32TAmb)
  [sTmIn_X_s32ClimtRcirc] -> SM3_Ki/6(sTmIn_X_s32ClimtRcirc)
  [sTmComprCtrl_D_u8HvacFlowLevel] -> SM3_Ki/7(sTmComprCtrl_D_u8HvacFlowLevel)
  [sTmSigProces_D_u8BattThermReq] -> SM3_Ki/8(sTmSigProces_D_u8BattThermReq)
  [sTmSigProces_D_u8HvBattCoolgReq] -> SM3_Ki/9(sTmSigProces_D_u8HvBattCoolgReq)
  [SM1Error] -> SM3_Kp/1(SM1Error)
  [SM2Error] -> SM3_Kp/2(SM2Error)
  [sTmIn_D_u8DCChrgSt] -> SM3_Kp/3(sTmIn_D_u8DCChrgSt)
  [sTmIn_D_u8HeatPump] -> SM3_Kp/4(sTmIn_D_u8HeatPump)
  [sTmSigProces_Te_s32TAmb] -> SM3_Kp/5(sTmSigProces_Te_s32TAmb)
  [sTmIn_X_s32ClimtRcirc] -> SM3_Kp/6(sTmIn_X_s32ClimtRcirc)
  [sTmComprCtrl_D_u8HvacFlowLevel] -> SM3_Kp/7(sTmComprCtrl_D_u8HvacFlowLevel)
  [sTmSigProces_D_u8BattThermReq] -> SM3_Kp/8(sTmSigProces_D_u8BattThermReq)
  [sTmSigProces_D_u8HvBattCoolgReq] -> SM3_Kp/9(sTmSigProces_D_u8HvBattCoolgReq)
  sTmSigProces_Te_s32EvapFanReqRamp/1 -> [sTmSigProces_Te_s32EvapFanReqRamp]
  sTmDiag_D_u8TeEvapFltSt/1 -> [sTmDiag_D_u8TeEvapFltSt]
  sTmIn_D_u8DCChrgSt/1 -> [sTmIn_D_u8DCChrgSt]
  sTmIn_D_u8HeatPump/1 -> [sTmIn_D_u8HeatPump]
  sTmSigProces_Te_s32TAmb/1 -> [sTmSigProces_Te_s32TAmb]
  sTmIn_Te_s32BattHv/1 -> [sTmIn_Te_s32BattHv]
  sTmIn_Te_s32HvBattCooltTReq/1 -> Saturation/1
  sTmIn_X_s32ClimtRcirc/1 -> [sTmIn_X_s32ClimtRcirc]
  sTmComprCtrl_D_u8HvacFlowLevel/1 -> [sTmComprCtrl_D_u8HvacFlowLevel]
  sTmSigProces_D_u8BattThermReq/1 -> [sTmSigProces_D_u8BattThermReq]
  sTmSigProces_D_u8HvBattCoolgReq/1 -> [sTmSigProces_D_u8HvBattCoolgReq]
  sTmSigProces_Te_s32EvapFanFilter/1 -> [sTmSigProces_Te_s32EvapFanFilter]
  sTmSigProces_Te_s32HvBattCooltTFilter/1 -> [sTmSigProces_Te_s32HvBattCooltTFilter]
  sTmSigProces_Te_s32SatLp/1 -> [sTmSigProces_Te_s32SatLp]
  xTmComprCtrl_B_CompOnReqCompOn/1 -> [xTmComprCtrl_B_CompOnReqCompOn]
  [SM1Error] -> ID26262_SM3FF/1(sTmIn_Te_s32HvBattCooltTReq)
  [sTmSigProces_Te_s32EvapFanReqRamp] -> ID26262_SM3FF/2(sTmSigProces_Te_s32EvapFanReqRamp)
  [sTmIn_D_u8DCChrgSt] -> ID26262_SM3FF/3(sTmIn_D_u8DCChrgSt)
  [sTmSigProces_Te_s32TAmb] -> ID26262_SM3FF/4(sTmSigProces_Te_s32TAmb)
  [sTmIn_Te_s32BattHv] -> ID26262_SM3FF/5(sTmIn_Te_s32BattHv)
  [sTmIn_X_s32ClimtRcirc] -> ID26262_SM3FF/6(sTmIn_X_s32ClimtRcirc)
  [sTmComprCtrl_D_u8HvacFlowLevel] -> ID26262_SM3FF/7(sTmComprCtrl_D_u8HvacFlowLevel)
  [sTmSigProces_D_u8HvBattCoolgReq] -> ID26262_SM3FF/8(sTmSigProces_D_u8HvBattCoolgReq)
  SM3SM1Error/1(rTmComprCtrl_Te_s32TempError) -> [SM1Error]
  [sTmSigProces_Te_s32EvapFanReqRamp] -> ID26263_SM3Error/1(sTmSigProces_Te_s32EvapFanReqRamp)
  [sTmIn_D_u8HeatPump] -> ID26263_SM3Error/2(sTmIn_D_u8HeatPump)
  [sTmIn_Te_s32HvBattCooltTReq] -> ID26263_SM3Error/3(sTmIn_Te_s32HvBattCooltTReq)
  [sTmSigProces_D_u8HvBattCoolgReq] -> ID26263_SM3Error/4(sTmSigProces_D_u8HvBattCoolgReq)
  [sTmSigProces_Te_s32EvapFanFilter] -> ID26263_SM3Error/5(sTmSigProces_Te_s32EvapFanFilter)
  [sTmSigProces_Te_s32HvBattCooltTFilter] -> ID26263_SM3Error/6(sTmSigProces_Te_s32HvBattCooltTFilter)
  [xTmComprCtrl_B_CompOnReqCompOn] -> ID26262_SM3FF/9(xTmComprCtrl_B_CompOnReqCompOn)
  ID26262_SM3FF/1(SM3FF) -> [rTmComprCtrl_n_u16ComprRpmFF]
  SM3_Kp/1(SM3Kp) -> [rTmComprCtrl_n_u16ComprRpmKp]
  [sTmSigProces_D_u8HvBattCoolgReq] -> Compare To Constant4/1
  Compare To Constant4/1 -> Switch2/2
  Switch2/1 -> [rTmComprCtrl_Te_s32UpErrStop]
  [sTmSigProces_D_u8HvBattCoolgReq] -> Compare To Constant5/1
  Switch3/1 -> [rTmComprCtrl_Te_s32LowErrStop]
  Compare To Constant5/1 -> Switch3/2
  Compare To Constant6/1 -> Switch4/2
  Switch4/1 -> [rTmComprCtrl_n_i16KpUpLimit]
  [sTmSigProces_D_u8HvBattCoolgReq] -> Compare To Constant6/1
  [sTmSigProces_D_u8HvBattCoolgReq] -> Compare To Constant7/1
  Switch5/1 -> [rTmComprCtrl_n_i16KpLowLimit]
  Compare To Constant7/1 -> Switch5/2
  Compare To Constant11/1 -> Switch9/2
  Switch7/1 -> [rTmComprCtrl_n_i16KiLowLimit]
  Switch9/1 -> [rTmComprCtrl_t_u16PIPeriod]
  Compare To Constant9/1 -> Switch7/2
  [sTmSigProces_D_u8HvBattCoolgReq] -> Compare To Constant11/1
  [sTmSigProces_D_u8HvBattCoolgReq] -> Compare To Constant9/1
  [sTmSigProces_D_u8HvBattCoolgReq] -> Compare To Constant8/1
  Switch6/1 -> [rTmComprCtrl_n_i16KiUpLimit]
  Constant33/1 -> [rTmComprCtrl_n_u16DisOverrideValue]
  Compare To Constant8/1 -> Switch6/2
  Constant34/1 -> [xTmComprCtrl_B_Enable]
  Constant2/1 -> Switch9/3
  Constant1/1 -> Switch9/1
  Constant/1 -> Switch2/1
  Constant13/1 -> Switch3/1
  Constant29/1 -> Switch4/1
  Constant30/1 -> Switch5/1
  Constant31/1 -> Switch6/1
  Constant32/1 -> Switch7/1
  Constant35/1 -> Switch2/3
  Constant36/1 -> Switch3/3
  Constant37/1 -> Switch4/3
  Constant38/1 -> Switch5/3
  Constant39/1 -> Switch6/3
  Constant40/1 -> Switch7/3
  SM3_Ki/1(SM3Ki) -> [rTmComprCtrl_n_u16ComprRpmKi]
  [xTmComprCtrl_B_ModeChanged] -> ID26263_SM3Error/7(xTmComprCtrl_B_ModeChanged)
  xTmComprCtrl_B_ModeChanged/1 -> [xTmComprCtrl_B_ModeChanged]
  [yTmRefriModeMgr_B_CoolOCRMode] -> SM3SM2Error/5(yTmRefriModeMgr_B_CoolOCRMode)
  yTmRefriModeMgr_B_CoolOCRMode/1 -> [yTmRefriModeMgr_B_CoolOCRMode]
  Saturation/1 -> [sTmIn_Te_s32HvBattCooltTReq]
  [sTmIn_D_u8HeatPump] -> ID26262_SM3FF/10(sTmIn_D_u8HeatPump)
  [rTmComprCtrl_n_u16ComprRpmKi] -> rSM3SM23_n_u16ComprRpmKi/1
  [rTmComprCtrl_Te_s32UpErrStop] -> rSM3SM23_Te_s32UpErrStop/1
  [rTmComprCtrl_n_u16ComprRpmFF] -> rSM3SM23_n_u16ComprRpmFF/1
  [rTmComprCtrl_n_u16DisOverrideValue] -> rSM3SM23_n_u16DisOverrideValue/1
  [rTmComprCtrl_t_u16PIPeriod] -> rSM3SM23_t_u16PIPeriod/1
  [xTmComprCtrl_B_Enable] -> xSM3SM23_B_Enable/1
  [rTmComprCtrl_n_u16ComprRpmKp] -> rSM3SM23_n_u16ComprRpmKp/1
  [rTmComprCtrl_Te_s32LowErrStop] -> rSM3SM23_Te_s32LowErrStop/1
  [rTmComprCtrl_n_i16KpUpLimit] -> rSM3SM23_n_i16KpUpLimit/1
  [rTmComprCtrl_n_i16KpLowLimit] -> rSM3SM23_n_i16KpLowLimit/1
  [rTmComprCtrl_n_i16KiUpLimit] -> rSM3SM23_n_i16KiUpLimit/1
  [rTmComprCtrl_n_i16KiLowLimit] -> rSM3SM23_n_i16KiLowLimit/1
  [rTmComprCtrl_Te_s32TempError] -> rSM3SM23_Te_s32TempError/1

== system ScriptDemo/Create/createMerge/Before/SM4 ==
  sTmSigProces_Te_s32HeatrAirTReqRamp : Inport  OutDataTypeStr=single
  sTmSigProces_Te_s32HvacHexAirTFilter : Inport  Port=2  OutDataTypeStr=single
  sTmSigProces_Te_s32TAmb : Inport  Port=3  OutDataTypeStr=single
  sTmSigProces_Te_s32SatHp : Inport  Port=4  OutDataTypeStr=single
  sTmComprCtrl_D_u8HvacFlowLevel : Inport  Port=5  OutDataTypeStr=uint8
  xTmComprCtrl_B_CompOnReqCompOn : Inport  Port=6  OutDataTypeStr=boolean
  yTmHvchCtrl_B_HpcPtcEnad : Inport  Port=7  OutDataTypeStr=boolean
  sTmSigProces_Te_s32TempInlet : Inport  Port=8  OutDataTypeStr=single
  yTmRefriModeMgr_B_HeatModeInCycle : Inport  Port=9  OutDataTypeStr=boolean
  Action Port : ActionPort
  Constant : Constant  Value=cTmComprCtrl_n_i16SM4CmpHeatKpMax  OutDataTypeStr=int16
  Constant15 : Constant  Value=cTmComprCtrl_Te_s32ErrCmpPIContinueHeatL  OutDataTypeStr=single
  Constant16 : Constant  Value=cTmComprCtrl_n_i16SM4CmpHeatKiMin  OutDataTypeStr=int16
  Constant2 : Constant  Value=cTmComprCtrl_n_u16CompMinRpm
  Constant6 : Constant  Value=cTmComprCtrl_t_u16SM4CmpHeatPIPeriod  OutDataTypeStr=uint16
  Constant7 : Constant  Value=cTmComprCtrl_n_i16SM4CmpHeatKpMin  OutDataTypeStr=int16
  Constant8 : Constant  Value=cTmComprCtrl_Te_s32ErrCmpPIContinueHeatH  OutDataTypeStr=single
  Constant9 : Constant  Value=cTmComprCtrl_n_i16SM4CmpHeatKiMax  OutDataTypeStr=int16
  ID26259_SM4Error : Subsystem
  ID26297_SM4FF : Subsystem
  Logical Operator : Logic  Operator=NOT  AllPortsSameDT=off  OutDataTypeStr=boolean
  SM24FFEnable : Subsystem
  SM4_Ki : Subsystem
  SM4_Kp : Subsystem
  rSM4_n_u16DisOverrideValue : Outport  OutDataTypeStr=uint16
  rSM4_t_u16PIPeriod : Outport  Port=2  OutDataTypeStr=uint16
  rSM4_Te_s32UpErrStop : Outport  Port=3  OutDataTypeStr=single
  rSM4_n_u16ComprRpmFF : Outport  Port=4  OutDataTypeStr=uint16
  rSM4_n_u16ComprRpmKp : Outport  Port=5  OutDataTypeStr=uint16
  rSM4_Te_s32LowErrStop : Outport  Port=6  OutDataTypeStr=single
  rSM4_n_i16KpUpLimit : Outport  Port=7  OutDataTypeStr=int16
  rSM4_n_i16KpLowLimit : Outport  Port=8  OutDataTypeStr=int16
  rSM4_n_i16KiUpLimit : Outport  Port=9  OutDataTypeStr=int16
  rSM4_n_i16KiLowLimit : Outport  Port=10  OutDataTypeStr=int16
  xSM4_B_Enable : Outport  Port=11  OutDataTypeStr=boolean
  rSM4_n_u16ComprRpmKi : Outport  Port=12  OutDataTypeStr=uint16
  rSM4_Te_s32TempError : Outport  Port=13  OutDataTypeStr=single
  wires:
  ID26259_SM4Error/1(rTmComprCtrl_Te_s32TempError) -> [rTmComprCtrl_Te_s32TempError]
  [sTmSigProces_Te_s32SatHp] -> ID26259_SM4Error/1(sTmSigProces_Te_s32SatHp)
  [yTmHvchCtrl_B_HpcPtcEnad] -> ID26259_SM4Error/2(yTmHvchCtrl_B_HpcPtcEnad)
  [sTmSigProces_Te_s32HeatrAirTReqRamp] -> ID26259_SM4Error/3(sTmSigProces_Te_s32HeatrAirTReqRamp)
  [sTmSigProces_Te_s32HvacHexAirTFilter] -> ID26259_SM4Error/4(sTmSigProces_Te_s32HvacHexAirTFilter)
  sTmSigProces_Te_s32HeatrAirTReqRamp/1 -> [sTmSigProces_Te_s32HeatrAirTReqRamp]
  sTmSigProces_Te_s32HvacHexAirTFilter/1 -> [sTmSigProces_Te_s32HvacHexAirTFilter]
  sTmSigProces_Te_s32TAmb/1 -> [sTmSigProces_Te_s32TAmb]
  sTmSigProces_Te_s32SatHp/1 -> [sTmSigProces_Te_s32SatHp]
  sTmComprCtrl_D_u8HvacFlowLevel/1 -> [sTmComprCtrl_D_u8HvacFlowLevel]
  xTmComprCtrl_B_CompOnReqCompOn/1 -> [xTmComprCtrl_B_CompOnReqCompOn]
  yTmHvchCtrl_B_HpcPtcEnad/1 -> [yTmHvchCtrl_B_HpcPtcEnad]
  [xTmComprCtrl_B_CompOnReqCompOn] -> SM24FFEnable/1(xTmComprCtrl_B_CompOnReqCompOn)
  SM24FFEnable/1(SM4FFEnable_B_SM4FFEnable) -> [SM4FFEnable_B_SM4FFEnable]
  [SM4FFEnable_B_SM4FFEnable] -> ID26297_SM4FF/Enable
  Logical Operator/1 -> [xTmComprCtrl_B_Enable]
  Constant2/1 -> [rTmComprCtrl_n_u16DisOverrideValue]
  Constant6/1 -> [rTmComprCtrl_t_u16PIPeriod]
  Constant15/1 -> [rTmComprCtrl_Te_s32LowErrStop]
  Constant/1 -> [rTmComprCtrl_n_i16KpUpLimit]
  Constant8/1 -> [rTmComprCtrl_Te_s32UpErrStop]
  Constant7/1 -> [rTmComprCtrl_n_i16KpLowLimit]
  Constant16/1 -> [rTmComprCtrl_n_i16KiLowLimit]
  Constant9/1 -> [rTmComprCtrl_n_i16KiUpLimit]
  ID26297_SM4FF/1(SM4FF) -> [rTmComprCtrl_n_u16ComprRpmFF]
  SM4_Kp/1(SM4Kp) -> [rTmComprCtrl_n_u16ComprRpmKp]
  SM4_Ki/1(SM4Ki) -> [rTmComprCtrl_n_u16ComprRpmKi]
  sTmSigProces_Te_s32TempInlet/1 -> [sTmSigProces_Te_s32TempInlet]
  [sTmComprCtrl_D_u8HvacFlowLevel] -> ID26297_SM4FF/1(sTmComprCtrl_D_u8HvacFlowLevel)
  [sTmSigProces_Te_s32TempInlet] -> ID26297_SM4FF/2(sTmSigProces_Te_s32TempInlet)
  [sTmSigProces_Te_s32HeatrAirTReqRamp] -> ID26297_SM4FF/3(sTmSigProces_Te_s32HeatrAirTReqRamp)
  [sTmSigProces_Te_s32TAmb] -> ID26297_SM4FF/4(sTmSigProces_Te_s32TAmb)
  [sTmComprCtrl_D_u8HvacFlowLevel] -> SM4_Ki/1(sTmComprCtrl_D_u8HvacFlowLevel)
  [sTmSigProces_Te_s32TAmb] -> SM4_Ki/2(sTmSigProces_Te_s32TAmb)
  [rTmComprCtrl_Te_s32TempError] -> SM4_Ki/3(rTmComprCtrl_Te_s32TempError)
  [sTmComprCtrl_D_u8HvacFlowLevel] -> SM4_Kp/1(sTmComprCtrl_D_u8HvacFlowLevel)
  [sTmSigProces_Te_s32TAmb] -> SM4_Kp/2(sTmSigProces_Te_s32TAmb)
  [rTmComprCtrl_Te_s32TempError] -> SM4_Kp/3(rTmComprCtrl_Te_s32TempError)
  [yTmRefriModeMgr_B_HeatModeInCycle] -> Logical Operator/1
  yTmRefriModeMgr_B_HeatModeInCycle/1 -> [yTmRefriModeMgr_B_HeatModeInCycle]
  [rTmComprCtrl_n_u16DisOverrideValue] -> rSM4_n_u16DisOverrideValue/1
  [rTmComprCtrl_t_u16PIPeriod] -> rSM4_t_u16PIPeriod/1
  [rTmComprCtrl_Te_s32UpErrStop] -> rSM4_Te_s32UpErrStop/1
  [rTmComprCtrl_n_u16ComprRpmFF] -> rSM4_n_u16ComprRpmFF/1
  [rTmComprCtrl_n_u16ComprRpmKp] -> rSM4_n_u16ComprRpmKp/1
  [rTmComprCtrl_Te_s32LowErrStop] -> rSM4_Te_s32LowErrStop/1
  [rTmComprCtrl_n_i16KpUpLimit] -> rSM4_n_i16KpUpLimit/1
  [rTmComprCtrl_n_i16KpLowLimit] -> rSM4_n_i16KpLowLimit/1
  [rTmComprCtrl_n_i16KiUpLimit] -> rSM4_n_i16KiUpLimit/1
  [rTmComprCtrl_n_i16KiLowLimit] -> rSM4_n_i16KiLowLimit/1
  [xTmComprCtrl_B_Enable] -> xSM4_B_Enable/1
  [rTmComprCtrl_n_u16ComprRpmKi] -> rSM4_n_u16ComprRpmKi/1
  [rTmComprCtrl_Te_s32TempError] -> rSM4_Te_s32TempError/1

== system ScriptDemo/Create/createMerge/Before/SM5 ==
  note: 20240303
  note: sTmSigProces_Te_s32HvBattCooltTFilter-->sTmSigProces_Te_s32SatLp
  note: sTmIn_Te_s32AmbTEstimd-->sTmSigProces_Te_s32SatLp
  sTmSigProces_Te_s32SatLp : Inport  OutDataTypeStr=single
  sTmSigProces_Te_s32HvBattCooltTFilter : Inport  Port=2  OutDataTypeStr=single
  sTmSigProces_Te_s32HeatrAirTReqRamp : Inport  Port=3  OutDataTypeStr=single
  sTmSigProces_Te_s32HvacHexAirTFilter : Inport  Port=4  OutDataTypeStr=single
  sTmSigProces_Te_s32TempInlet : Inport  Port=5  OutDataTypeStr=single
  sTmSigProces_Te_s32SatHp : Inport  Port=6  OutDataTypeStr=single
  sTmComprCtrl_D_u8HvacFlowLevel : Inport  Port=7  OutDataTypeStr=uint8
  xTmComprCtrl_B_CompOnReqCompOn : Inport  Port=8  OutDataTypeStr=boolean
  yTmHvchCtrl_B_HpcPtcEnad : Inport  Port=9  OutDataTypeStr=boolean
  Action Port : ActionPort
  Constant : Constant  Value=cTmComprCtrl_n_i16SM5CmpHeatKpMax  OutDataTypeStr=int16
  Constant1 : Constant  OutDataTypeStr=boolean
  Constant15 : Constant  Value=cTmComprCtrl_Te_s32ErrCmpPIContinueHeatL  OutDataTypeStr=single
  Constant16 : Constant  Value=cTmComprCtrl_n_i16SM5CmpHeatKiMin  OutDataTypeStr=int16
  Constant17 : Constant  Value=0  OutDataTypeStr=uint16
  Constant6 : Constant  Value=cTmComprCtrl_t_u16SM5CmpHeatPIPeriod  OutDataTypeStr=uint16
  Constant7 : Constant  Value=cTmComprCtrl_n_i16SM5CmpHeatKpMin  OutDataTypeStr=int16
  Constant8 : Constant  Value=cTmComprCtrl_Te_s32ErrCmpPIContinueHeatH  OutDataTypeStr=single
  Constant9 : Constant  Value=cTmComprCtrl_n_i16SM5CmpHeatKiMax  OutDataTypeStr=int16
  ID26291_SM5FF : Subsystem
  ID26293_SM5Error : Subsystem
  SM5FFEnable : Subsystem
  SM5_Ki : Subsystem
  SM5_Kp : Subsystem
  Terminator1 : Terminator
  rSM5_n_u16DisOverrideValue : Outport  OutDataTypeStr=uint16
  rSM5_t_u16PIPeriod : Outport  Port=2  OutDataTypeStr=uint16
  rSM5_Te_s32UpErrStop : Outport  Port=3  OutDataTypeStr=single
  rSM5_n_u16ComprRpmFF : Outport  Port=4  OutDataTypeStr=uint16
  rSM5_n_u16ComprRpmKp : Outport  Port=5  OutDataTypeStr=uint16
  rSM5_Te_s32LowErrStop : Outport  Port=6  OutDataTypeStr=single
  rSM5_n_i16KpUpLimit : Outport  Port=7  OutDataTypeStr=int16
  rSM5_n_i16KpLowLimit : Outport  Port=8  OutDataTypeStr=int16
  rSM5_n_i16KiUpLimit : Outport  Port=9  OutDataTypeStr=int16
  rSM5_n_i16KiLowLimit : Outport  Port=10  OutDataTypeStr=int16
  xSM5_B_Enable : Outport  Port=11  OutDataTypeStr=boolean
  rSM5_n_u16ComprRpmKi : Outport  Port=12  OutDataTypeStr=uint16
  rSM5_Te_s32TempError : Outport  Port=13  OutDataTypeStr=single
  wires:
  ID26293_SM5Error/1(rTmComprCtrl_Te_s32TempError) -> [rTmComprCtrl_Te_s32TempError]
  [sTmSigProces_Te_s32SatHp] -> ID26293_SM5Error/1(sTmSigProces_Te_s32SatHp)
  [yTmHvchCtrl_B_HpcPtcEnad] -> ID26293_SM5Error/2(yTmHvchCtrl_B_HpcPtcEnad)
  [sTmSigProces_Te_s32HeatrAirTReqRamp] -> ID26293_SM5Error/3(sTmSigProces_Te_s32HeatrAirTReqRamp)
  [sTmSigProces_Te_s32HvacHexAirTFilter] -> ID26293_SM5Error/4(sTmSigProces_Te_s32HvacHexAirTFilter)
  sTmSigProces_Te_s32SatLp/1 -> [sTmSigProces_Te_s32SatLp]
  sTmSigProces_Te_s32HvBattCooltTFilter/1 -> Terminator1/1
  sTmSigProces_Te_s32HeatrAirTReqRamp/1 -> [sTmSigProces_Te_s32HeatrAirTReqRamp]
  sTmSigProces_Te_s32HvacHexAirTFilter/1 -> [sTmSigProces_Te_s32HvacHexAirTFilter]
  sTmSigProces_Te_s32TempInlet/1 -> [sTmSigProces_Te_s32TempInlet]
  sTmSigProces_Te_s32SatHp/1 -> [sTmSigProces_Te_s32SatHp]
  sTmComprCtrl_D_u8HvacFlowLevel/1 -> [sTmComprCtrl_D_u8HvacFlowLevel]
  xTmComprCtrl_B_CompOnReqCompOn/1 -> [xTmComprCtrl_B_CompOnReqCompOn]
  yTmHvchCtrl_B_HpcPtcEnad/1 -> [yTmHvchCtrl_B_HpcPtcEnad]
  [xTmComprCtrl_B_CompOnReqCompOn] -> SM5FFEnable/1(xTmComprCtrl_B_CompOnReqCompOn)
  SM5FFEnable/1(SM5FFEnable_B_SM5FFEnable) -> [SM4FFEnable_B_SM4FFEnable]
  [SM4FFEnable_B_SM4FFEnable] -> ID26291_SM5FF/Enable
  ID26291_SM5FF/1(SM5FF) -> [rTmComprCtrl_n_u16ComprRpmFF]
  SM5_Kp/1(SM5Kp) -> [rTmComprCtrl_n_u16ComprRpmKp]
  SM5_Ki/1(SM5Ki) -> [rTmComprCtrl_n_u16ComprRpmKi]
  Constant1/1 -> [xTmComprCtrl_B_Enable]
  Constant16/1 -> [rTmComprCtrl_n_i16KiLowLimit]
  Constant9/1 -> [rTmComprCtrl_n_i16KiUpLimit]
  Constant7/1 -> [rTmComprCtrl_n_i16KpLowLimit]
  Constant8/1 -> [rTmComprCtrl_Te_s32UpErrStop]
  Constant/1 -> [rTmComprCtrl_n_i16KpUpLimit]
  Constant15/1 -> [rTmComprCtrl_Te_s32LowErrStop]
  Constant17/1 -> [rTmComprCtrl_n_u16DisOverrideValue]
  [sTmComprCtrl_D_u8HvacFlowLevel] -> ID26291_SM5FF/1(sTmComprCtrl_D_u8HvacFlowLevel)
  [sTmSigProces_Te_s32TempInlet] -> ID26291_SM5FF/2(sTmSigProces_Te_s32TempInlet)
  [sTmSigProces_Te_s32HeatrAirTReqRamp] -> ID26291_SM5FF/3(sTmSigProces_Te_s32HeatrAirTReqRamp)
  [sTmSigProces_Te_s32SatLp] -> ID26291_SM5FF/4(sTmSigProces_Te_s32SatLp)
  [sTmComprCtrl_D_u8HvacFlowLevel] -> SM5_Ki/1(sTmComprCtrl_D_u8HvacFlowLevel)
  [sTmSigProces_Te_s32SatLp] -> SM5_Ki/2(sTmSigProces_Te_s32SatLp)
  [rTmComprCtrl_Te_s32TempError] -> SM5_Ki/3(rTmComprCtrl_Te_s32TempError)
  [sTmComprCtrl_D_u8HvacFlowLevel] -> SM5_Kp/1(sTmComprCtrl_D_u8HvacFlowLevel)
  [sTmSigProces_Te_s32SatLp] -> SM5_Kp/2(sTmSigProces_Te_s32SatLp)
  [rTmComprCtrl_Te_s32TempError] -> SM5_Kp/3(rTmComprCtrl_Te_s32TempError)
  Constant6/1 -> [rTmComprCtrl_t_u16PIPeriod]
  [rTmComprCtrl_n_u16DisOverrideValue] -> rSM5_n_u16DisOverrideValue/1
  [rTmComprCtrl_t_u16PIPeriod] -> rSM5_t_u16PIPeriod/1
  [rTmComprCtrl_Te_s32UpErrStop] -> rSM5_Te_s32UpErrStop/1
  [rTmComprCtrl_n_u16ComprRpmFF] -> rSM5_n_u16ComprRpmFF/1
  [rTmComprCtrl_n_u16ComprRpmKp] -> rSM5_n_u16ComprRpmKp/1
  [rTmComprCtrl_Te_s32LowErrStop] -> rSM5_Te_s32LowErrStop/1
  [rTmComprCtrl_n_i16KpUpLimit] -> rSM5_n_i16KpUpLimit/1
  [rTmComprCtrl_n_i16KpLowLimit] -> rSM5_n_i16KpLowLimit/1
  [rTmComprCtrl_n_i16KiUpLimit] -> rSM5_n_i16KiUpLimit/1
  [rTmComprCtrl_n_i16KiLowLimit] -> rSM5_n_i16KiLowLimit/1
  [xTmComprCtrl_B_Enable] -> xSM5_B_Enable/1
  [rTmComprCtrl_n_u16ComprRpmKi] -> rSM5_n_u16ComprRpmKi/1
  [rTmComprCtrl_Te_s32TempError] -> rSM5_Te_s32TempError/1
